simulink library "se2a_actuators_lib"  (R2018b)
settings: Solver=VariableStepAuto  StartTime=0.0  StopTime=10.0  RelTol=1e-3
undefined symbols (not defined in the file or in its folder): aileron, elevator, engine_params, htp, LADs, rudder
libraries: unit_conversions_lib x7, actuators_lib x5
settings Model: Creator=Ybeyer  LastModifiedBy=yannic
settings SFSimCC: SimUseLocalCustomCode=off
settings RTWCC: RTWUseLocalCustomCode=off
settings CodeAppCC: StateflowObjectComments=on

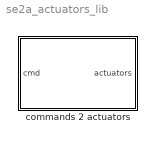
== system se2a_actuators_lib ==
  commands 2 actuators : Subsystem  mask{aileron=aileron, elevator=elevator, rudder=rudder, lads=LADs, engines=engine_params, htp_trim=htp}
      mask prompts: aileron "Aileron parameters"; elevator "Elevator parameters"; rudder "Rudder parameters"; lads "Load alleviation devices (LADs) parameters"; engines "Engines parameters"; htp_trim "Trimmable horizontal tailplane (htp) parameters"
      mask DialogControl DescGroupVar Prompt: SE2A Actuator Dynamics
      mask DialogControl DescTextVar Prompt: Input commands are defined as bus.

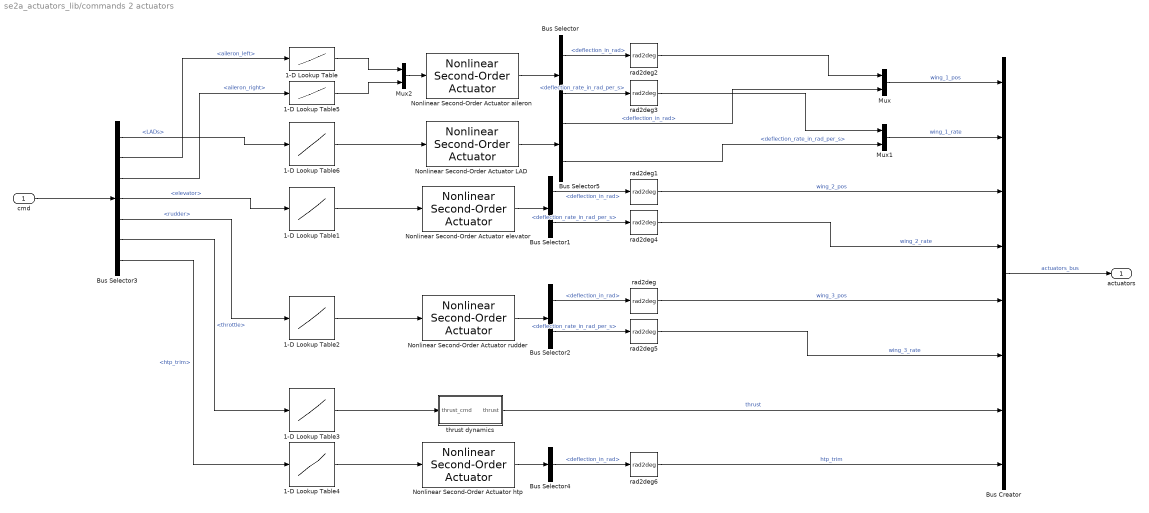
== system se2a_actuators_lib/commands 2 actuators ==
  cmd : Inport
  1-D Lookup Table : Lookup_n-D  NumberOfTableDimensions=1  BreakpointsForDimension1=[-1,1]  Table=[aileron.defl_min,aileron.defl_max]  ExtrapMethod=Clip  InternalRulePriority=Speed  RndMeth=Simplest  InputSameDT=on
  1-D Lookup Table1 : Lookup_n-D  NumberOfTableDimensions=1  BreakpointsForDimension1=[-1,1]  Table=[elevator.defl_min,elevator.defl_max]  ExtrapMethod=Clip  InternalRulePriority=Speed  RndMeth=Simplest  InputSameDT=on
  1-D Lookup Table2 : Lookup_n-D  NumberOfTableDimensions=1  BreakpointsForDimension1=[-1,1]  Table=[rudder.defl_min,rudder.defl_max]  ExtrapMethod=Clip  InternalRulePriority=Speed  RndMeth=Simplest  InputSameDT=on
  1-D Lookup Table3 : Lookup_n-D  NumberOfTableDimensions=1  BreakpointsForDimension1=[0,1]  Table=[0,engines.thrust_max]  ExtrapMethod=Clip  InternalRulePriority=Speed  RndMeth=Simplest  InputSameDT=on
  1-D Lookup Table4 : Lookup_n-D  NumberOfTableDimensions=1  BreakpointsForDimension1=[-1,1]  Table=[htp_trim.defl_min,htp_trim.defl_max]  ExtrapMethod=Clip  InternalRulePriority=Speed  RndMeth=Simplest  InputSameDT=on
  1-D Lookup Table5 : Lookup_n-D  NumberOfTableDimensions=1  BreakpointsForDimension1=[-1,1]  Table=[aileron.defl_min,aileron.defl_max]  ExtrapMethod=Clip  InternalRulePriority=Speed  RndMeth=Simplest  InputSameDT=on
  1-D Lookup Table6 : Lookup_n-D  NumberOfTableDimensions=1  BreakpointsForDimension1=[-1,1]  Table=[lads.defl_min,lads.defl_max]  ExtrapMethod=Clip  InternalRulePriority=Speed  RndMeth=Simplest  InputSameDT=on
  Bus Creator : BusCreator  Inputs=8
  Bus Selector{,1..2,5} (4 alike) : BusSelector  OutputSignals=deflection_in_rad,deflection_rate_in_rad_per_s
  Bus Selector3 : BusSelector  OutputSignals=LADs,aileron_left,aileron_right,elevator,rudder,throttle,htp_trim
  Bus Selector4 : BusSelector  OutputSignals=deflection_in_rad
  Mux : Mux  Inputs=2
  Mux1 : Mux  Inputs=2
  Mux2 : Mux  Inputs=2
  Nonlinear Second-Order Actuator LAD : actuators_lib/Nonlinear Second-Order Actuator  omega=lads.omega  d=lads.D  A_max=lads.defl_max  A_min=lads.defl_min  dot_A_max=lads.defl_rate_max  dot_A_min=lads.defl_rate_min  A_0=0  dot_A_0=0
      settings: SourceProductName=LADAC
  Nonlinear Second-Order Actuator aileron : actuators_lib/Nonlinear Second-Order Actuator  omega=aileron.omega  d=aileron.D  A_max=aileron.defl_max  A_min=aileron.defl_min  dot_A_max=aileron.defl_rate_max  dot_A_min=aileron.defl_rate_min  A_0=0  dot_A_0=0
      settings: SourceProductName=LADAC
  Nonlinear Second-Order Actuator elevator : actuators_lib/Nonlinear Second-Order Actuator  omega=elevator.omega  d=elevator.D  A_max=elevator.defl_max  A_min=elevator.defl_min  dot_A_max=elevator.defl_rate_max  dot_A_min=elevator.defl_rate_min  A_0=0  dot_A_0=0
      settings: SourceProductName=LADAC
  Nonlinear Second-Order Actuator htp : actuators_lib/Nonlinear Second-Order Actuator  omega=htp_trim.omega  d=htp_trim.D  A_max=htp_trim.defl_max  A_min=htp_trim.defl_min  dot_A_max=htp_trim.defl_rate_max  dot_A_min=htp_trim.defl_rate_min  A_0=0  dot_A_0=0
      settings: SourceProductName=LADAC
  Nonlinear Second-Order Actuator rudder : actuators_lib/Nonlinear Second-Order Actuator  omega=rudder.omega  d=rudder.D  A_max=rudder.defl_max  A_min=rudder.defl_min  dot_A_max=rudder.defl_rate_max  dot_A_min=rudder.defl_rate_min  A_0=0  dot_A_0=0
      settings: SourceProductName=LADAC
  rad2deg{,1..6} (7 alike) : unit_conversions_lib/rad2deg
      settings: SourceProductName=LADAC
  thrust dynamics : Subsystem
  actuators : Outport
  wires:
  Bus Creator/1 -> actuators/1  "actuators_bus"
  Mux/1 -> Bus Creator/1  "wing_1_pos"
  rad2deg1/1 -> Bus Creator/3  "wing_2_pos"
  rad2deg/1 -> Bus Creator/5  "wing_3_pos"
  Bus Selector/1 -> rad2deg2/1  "<deflection_in_rad>"
  Nonlinear Second-Order Actuator elevator/1 -> Bus Selector1/1
  Nonlinear Second-Order Actuator rudder/1 -> Bus Selector2/1
  Nonlinear Second-Order Actuator aileron/1 -> Bus Selector/1
  Bus Selector1/1 -> rad2deg1/1  "<deflection_in_rad>"
  Bus Selector2/1 -> rad2deg/1  "<deflection_in_rad>"
  1-D Lookup Table/1 -> Mux2/1
  Bus Selector3/4 -> 1-D Lookup Table1/1  "<elevator>"
  1-D Lookup Table1/1 -> Nonlinear Second-Order Actuator elevator/1
  Bus Selector3/5 -> 1-D Lookup Table2/1  "<rudder>"
  1-D Lookup Table2/1 -> Nonlinear Second-Order Actuator rudder/1
  Bus Selector/2 -> rad2deg3/1  "<deflection_rate_in_rad_per_s>"
  Bus Selector1/2 -> rad2deg4/1  "<deflection_rate_in_rad_per_s>"
  Mux1/1 -> Bus Creator/2  "wing_1_rate"
  rad2deg4/1 -> Bus Creator/4  "wing_2_rate"
  Bus Selector2/2 -> rad2deg5/1  "<deflection_rate_in_rad_per_s>"
  rad2deg5/1 -> Bus Creator/6  "wing_3_rate"
  cmd/1 -> Bus Selector3/1
  Bus Selector3/1 -> 1-D Lookup Table6/1  "<LADs>"
  Bus Selector3/2 -> 1-D Lookup Table/1  "<aileron_left>"
  Bus Selector3/3 -> 1-D Lookup Table5/1  "<aileron_right>"
  Bus Selector3/6 -> 1-D Lookup Table3/1  "<throttle>"
  1-D Lookup Table3/1 -> thrust dynamics/1(thrust_cmd)
  thrust dynamics/1(thrust) -> Bus Creator/7  "thrust"
  Bus Selector3/7 -> 1-D Lookup Table4/1  "<htp_trim>"
  Bus Selector4/1 -> rad2deg6/1  "<deflection_in_rad>"
  Nonlinear Second-Order Actuator htp/1 -> Bus Selector4/1
  rad2deg6/1 -> Bus Creator/8  "htp_trim"
  1-D Lookup Table4/1 -> Nonlinear Second-Order Actuator htp/1
  1-D Lookup Table5/1 -> Mux2/2
  Mux2/1 -> Nonlinear Second-Order Actuator aileron/1
  rad2deg2/1 -> Mux/1
  rad2deg3/1 -> Mux1/1
  Bus Selector5/1 -> Mux/2  "<deflection_in_rad>"
  Bus Selector5/2 -> Mux1/2  "<deflection_rate_in_rad_per_s>"
  1-D Lookup Table6/1 -> Nonlinear Second-Order Actuator LAD/1
  Nonlinear Second-Order Actuator LAD/1 -> Bus Selector5/1

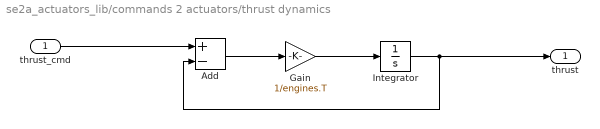
== system se2a_actuators_lib/commands 2 actuators/thrust dynamics ==
  thrust_cmd : Inport
  Add : Sum  Inputs=+-
  Gain : Gain  Gain=1/engines.T
  Integrator : Integrator
  thrust : Outport
  wires:
  Integrator/1 -> Add/2, thrust/1
  thrust_cmd/1 -> Add/1
  Add/1 -> Gain/1
  Gain/1 -> Integrator/1
